simulink model "lc_vsi"  (R2015a)
settings: Solver=ode23tb  StartTime=0.0  StopTime=0.1  FixedStep=1/20000/5  MaxStep=0.000005  RelTol=1e-3
values from neighbouring files (symbols this model uses):
  A = [-Rn/Ln -1/Ln; 1/Cn 0]    [LqgLtr.m]
  amp_dist = 0    [LqgLtr.m]
  amp_dist_2 = 0    [LqgLtr.m]
  amp_ref = 0.1    [LqgLtr.m]
  B = [-1/Ln; 0]    [LqgLtr.m]
  C = [1 0]    [LqgLtr.m]
  def = 2.4    [LqgLtr.m]
  freq_dist = 2*pi*60*5    (= 1884.95559215)    [LqgLtr.m]
  freq_dist_2 = 2*pi*60*7    (= 2638.93782902)    [LqgLtr.m]
  freq_ref = 377*5    (= 1885)    [LqgLtr.m]
  K = z*G*(z*eye(3)-(eye(3)-H*CDelay)*(PhiDelay-GammaDelay*G))^-1*H    [LqgLtr.m]
  step_1 = 0    [LqgLtr.m]
  step_2 = 1    [LqgLtr.m]
  t_step = 0.00005    (= 5e-05)    [LqgLtr.m]
  Vcc = 40    [LqgLtr.m]
libraries: powerlib_meascontrol x1
settings Model: Creator=Lucas  LastModifiedBy=brunopeixoto
settings SolverCC: AutoInsertRateTranBlk=on
settings OptimizationCC: InlineParams=on  UseDivisionForNetSlopeComputation=on  UseFloatMulNetSlope=on  InlineInvariantSignals=on  PassReuseOutputArgsAs=Individual arguments  ZeroExternalMemoryAtStartup=off  ZeroInternalMemoryAtStartup=off  NoFixptDivByZeroProtection=on  EfficientFloat2IntCast=on  OptimizeModelRefInitCode=on  LifeSpan=1
settings DebuggingCC: ReadBeforeWriteMsg=DisableAll  WriteAfterWriteMsg=DisableAll  WriteAfterReadMsg=DisableAll  UnderspecifiedInitializationDetection=Classic  MergeDetectMultiDrivingBlocksExec=none  SolverPrmCheckMsg=warning  ParameterTunabilityLossMsg=error  StateNameClashWarn=warning
settings HardwareCC: ProdLargestAtomicInteger=Long  ProdLargestAtomicFloat=Double  ProdIntDivRoundTo=Zero  ProdEndianess=LittleEndian  ProdHWDeviceType=ARM Compatible->ARM Cortex
settings RTWCC: SystemTargetFile=ert.tlc  TemplateMakefile=ert_default_tmf  Description=Embedded Coder  GenerateReport=on  IncludeHyperlinkInReport=on  LaunchReport=on  GenerateTraceInfo=on  GenerateTraceReport=on  GenerateTraceReportSl=on  GenerateTraceReportSf=on  GenerateTraceReportEml=on  GenerateCodeMetricsReport=on
settings CodeAppCC: ForceParamTrailComments=on  IgnoreCustomStorageClasses=off  OperatorAnnotations=on  SimulinkDataObjDesc=on  SFDataObjDesc=on  MATLABFcnDesc=on  CustomSymbolStrGlobalVar=rt$N$M  CustomSymbolStrType=$N$M  CustomSymbolStrFcn=$N$M$F  CustomSymbolStrMacro=$N$M  InsertBlockDesc=on  MATLABSourceComments=on
settings ERTTargetCC: MultiwordLength=256  ParMdlRefBuildCompliant=on  CompOptLevelCompliant=on  ConcurrentExecutionCompliant=on  IncludeMdlTerminateFcn=off  CombineSignalStateStructs=on  ERTFirstTimeCompliant=on  SupportComplex=off  SupportContinuousTime=off  SupportNonInlinedSFcns=on  SupportVariableSizeSignals=off  ModelStepFunctionPrototypeControlCompliant=on  CPPClassGenCompliant=on  ERTCustomFileTemplate=example_file_process.tlc  ERTFilePackagingFormat=CompactWithDataFile  ConvertIfToSwitch=on  SuppressUnreachableDefaultCases=on

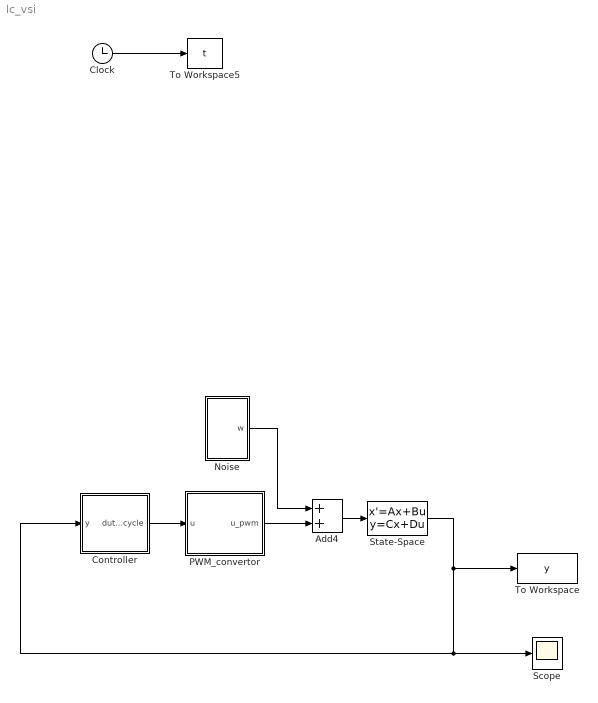
== system lc_vsi ==
  Add4 : Sum
  Clock : Clock
  Controller : Subsystem
  Noise : Subsystem
  PWM_convertor : Subsystem
  Scope : Scope
      settings: YMin=-0.80264  YMax=0.79195
  State-Space : StateSpace  A=A  B=B  C=C  D=0  X0=0
  To Workspace : ToWorkspace  VariableName=y  SampleTime=-1
  To Workspace5 : ToWorkspace  VariableName=t  SampleTime=-1
  wires:
  State-Space/1 -> To Workspace/1, Scope/1, Controller/1(y)
  Clock/1 -> To Workspace5/1
  Add4/1 -> State-Space/1
  Noise/1(w) -> Add4/1
  PWM_convertor/1(u_pwm) -> Add4/2
  Controller/1(duty_cycle) -> PWM_convertor/1(u)

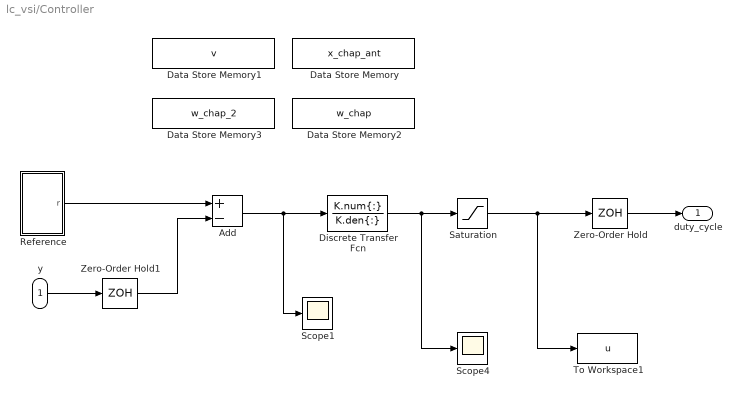
== system lc_vsi/Controller ==
  y : Inport
  Add : Sum  Inputs=+-
  Data Store Memory : DataStoreMemory  DataStoreName=x_chap_ant  ReadBeforeWriteMsg=warning  WriteAfterWriteMsg=warning  WriteAfterReadMsg=warning  InitialValue=[0; 0; 0; 0; 0; 0]  OutDataTypeStr=double
  Data Store Memory1 : DataStoreMemory  DataStoreName=v  ReadBeforeWriteMsg=warning  WriteAfterWriteMsg=warning  WriteAfterReadMsg=warning  InitialValue=[0]  OutDataTypeStr=double
  Data Store Memory2 : DataStoreMemory  DataStoreName=w_chap  ReadBeforeWriteMsg=warning  WriteAfterWriteMsg=warning  WriteAfterReadMsg=warning  OutDataTypeStr=double
  Data Store Memory3 : DataStoreMemory  DataStoreName=w_chap_2  ReadBeforeWriteMsg=warning  WriteAfterWriteMsg=warning  WriteAfterReadMsg=warning  OutDataTypeStr=double
  Discrete Transfer Fcn : DiscreteTransferFcn  Numerator=K.num{:}  Denominator=K.den{:}  SampleTime=1/20000
  Reference : Subsystem
  Saturation : Saturate  UpperLimit=40  LowerLimit=-40
  Scope1 : Scope
      settings: YMin=-0.54986  YMax=0.6619  SaveName=ScopeData6
  Scope4 : Scope
      settings: YMin=-635.16406  YMax=629.72455  SaveName=ScopeData4
  To Workspace1 : ToWorkspace  VariableName=u  SampleTime=-1
  Zero-Order Hold : ZeroOrderHold  SampleTime=1/20000
  Zero-Order Hold1 : ZeroOrderHold  SampleTime=1/20000
  duty_cycle : Outport
  wires:
  y/1 -> Zero-Order Hold1/1
  Saturation/1 -> Zero-Order Hold/1, To Workspace1/1
  Zero-Order Hold1/1 -> Add/2
  Add/1 -> Scope1/1, Discrete Transfer Fcn/1
  Discrete Transfer Fcn/1 -> Saturation/1, Scope4/1
  Zero-Order Hold/1 -> duty_cycle/1
  Reference/1(r) -> Add/1

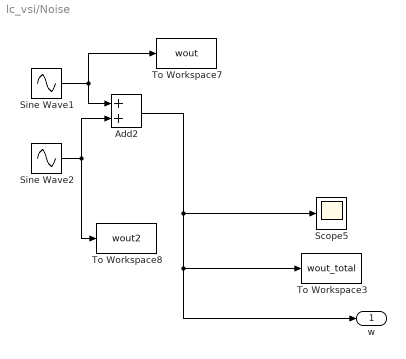
== system lc_vsi/Noise ==
  Add2 : Sum
  Scope5 : Scope
      settings: YMin=-0.1  YMax=0.175  SaveName=ScopeData5
  Sine Wave1 : Sin  Amplitude=amp_dist  Frequency=freq_dist  SampleTime=0
  Sine Wave2 : Sin  Amplitude=amp_dist_2  Frequency=freq_dist_2  SampleTime=0
  To Workspace3 : ToWorkspace  VariableName=wout_total  SampleTime=-1
  To Workspace7 : ToWorkspace  VariableName=wout  SampleTime=-1
  To Workspace8 : ToWorkspace  VariableName=wout2  SampleTime=-1
  w : Outport
  wires:
  Add2/1 -> w/1, To Workspace3/1, Scope5/1
  Sine Wave1/1 -> To Workspace7/1, Add2/1
  Sine Wave2/1 -> Add2/2, To Workspace8/1

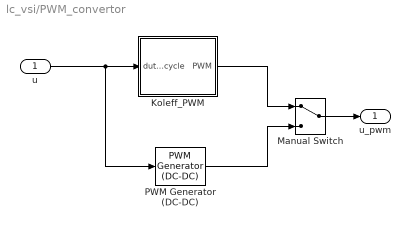
== system lc_vsi/PWM_convertor ==
  u : Inport
  Koleff_PWM : Subsystem
  Manual Switch : ManualSwitch
  PWM Generator (DC-DC) : powerlib_meascontrol/Pulse & Signal Generators/PWM Generator (DC-DC)  Fsw=5000  Ts=0
  u_pwm : Outport
  wires:
  u/1 -> PWM Generator (DC-DC)/1, Koleff_PWM/1(duty_cycle)
  Koleff_PWM/1(PWM) -> Manual Switch/1
  PWM Generator (DC-DC)/1 -> Manual Switch/2
  Manual Switch/1 -> u_pwm/1

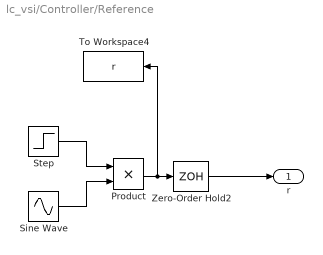
== system lc_vsi/Controller/Reference ==
  Product : Product
  Sine Wave : Sin  Amplitude=amp_ref  Frequency=freq_ref  Phase=def  SampleTime=0
  Step : Step  Time=t_step  Before=step_1  After=step_2  SampleTime=0
  To Workspace4 : ToWorkspace  VariableName=r  SampleTime=-1
  Zero-Order Hold2 : ZeroOrderHold  SampleTime=1/20000
  r : Outport
  wires:
  Product/1 -> To Workspace4/1, Zero-Order Hold2/1
  Sine Wave/1 -> Product/2
  Step/1 -> Product/1
  Zero-Order Hold2/1 -> r/1

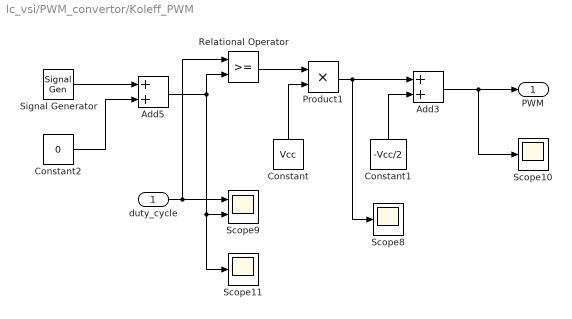
== system lc_vsi/PWM_convertor/Koleff_PWM ==
  duty_cycle : Inport
  Add3 : Sum
  Add5 : Sum
  Constant : Constant  Value=Vcc
  Constant1 : Constant  Value=-Vcc/2
  Constant2 : Constant  Value=0
  Product1 : Product
  Relational Operator : RelationalOperator  OutDataTypeStr=boolean
  Scope10 : Scope
      settings: YMin=-25.00000  YMax=25.00000
  Scope11 : Scope
      settings: YMin=-2.5  YMax=22.5  SaveName=ScopeData2
  Scope8 : Scope
      settings: YMin=-5.00000  YMax=45.00000  SaveName=ScopeData3
  Scope9 : Scope  NumInputPorts=2
      settings: YMin=-50.00000~-5  YMax=50.00000~5  SaveName=ScopeData5
  Signal Generator : SignalGenerator  WaveForm=sawtooth  Amplitude=40  Frequency=20000
  PWM : Outport
  wires:
  duty_cycle/1 -> Relational Operator/1, Scope9/1
  Add5/1 -> Scope9/2, Scope11/1, Relational Operator/2
  Constant2/1 -> Add5/2
  Signal Generator/1 -> Add5/1
  Product1/1 -> Add3/1, Scope8/1
  Constant1/1 -> Add3/2
  Constant/1 -> Product1/2
  Relational Operator/1 -> Product1/1
  Add3/1 -> PWM/1, Scope10/1
